simulink model "conmutador"  (Simulink 7.1)
settings: Solver=ode45  StartTime=0.0  StopTime=10000  RelTol=1e-3
values from neighbouring files (symbols this model uses):
  p = utilizacion(i)    [script_2x2.m]    (also in work.mat = 0.99)
libraries: simeventssink1 x8, simeventsrouting1 x8, simeventsqueue1 x4, simeventsgates1 x4, simeventsgenerators1 x4, simeventstiming1 x3, simeventsattributes1 x2, simeventsattributes2 x2, simeventsserver1 x2
settings Model: Creator=San  LastModifiedBy=EmP
settings DebuggingCC: SaveWithParameterizedLinksMsg=none  SignalResolutionControl=TryResolveAllWithWarning
settings GRTTargetCC: TargetFcnLib=ansi_tfl_tmw.mat
settings SimEventsCC: propLogEventsScheduled=0  propLogEventsExecuted=0  propLogDepartureEvents=0  propDisplayEventCalendar=0  propDiagAttribOutput=1  propDiagFcnCallOutput=1  propDiagStatOutput=0

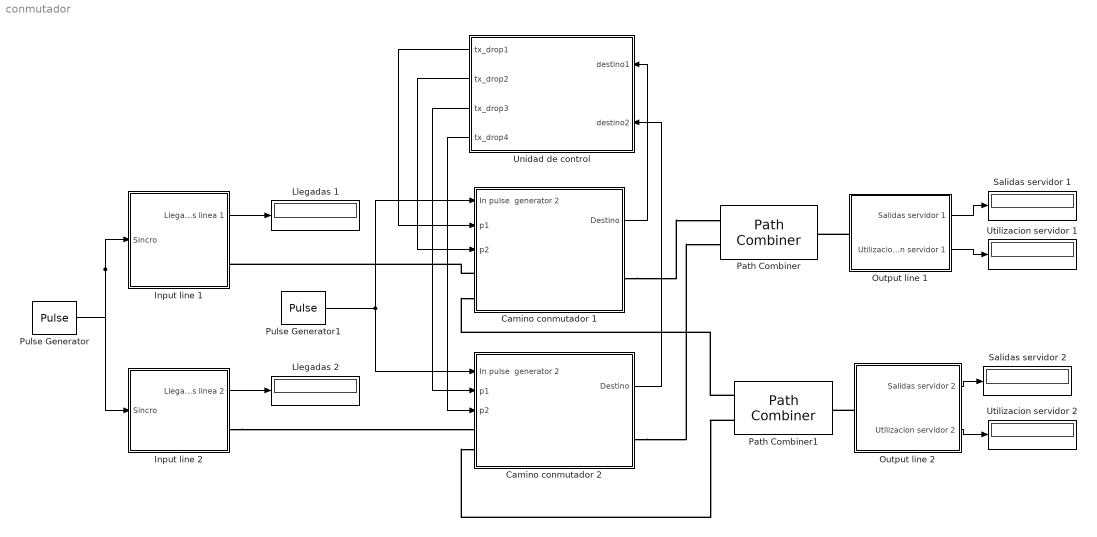
== system conmutador ==
  Camino conmutador 1 : Subsystem
  Camino conmutador 2 : Subsystem
  Input line 1 : Subsystem
  Input line 2 : Subsystem
  Llegadas 1 : Display
  Llegadas 2 : Display
  Output line 1 : Subsystem
  Output line 2 : Subsystem
  Path Combiner : simeventsrouting1/Path Combiner  Priority=1  SystemSampleTime=-1  NumberInputPorts=2  InputPortPrecedence=IN1 port  InitialSeed=45675  SpecifyEventPriority=off  PriorityPathCombinerPortPrecedenceSelection=4100  StatNumberDeparted=Off  StatLastArrivalPort=Off  EvaluatedNumPorts=2
  Path Combiner1 : simeventsrouting1/Path Combiner  Priority=1  SystemSampleTime=-1  NumberInputPorts=2  InputPortPrecedence=IN1 port  InitialSeed=45675  SpecifyEventPriority=off  PriorityPathCombinerPortPrecedenceSelection=4100  StatNumberDeparted=Off  StatLastArrivalPort=Off  EvaluatedNumPorts=2
  Pulse Generator : DiscretePulseGenerator  PulseType=Time based  Period=1  PulseWidth=50  SampleTime=1/10000
  Pulse Generator1 : DiscretePulseGenerator  PulseType=Time based  Period=1  PulseWidth=50  PhaseDelay=0.5  SampleTime=1/10000
  Salidas servidor 1 : Display
  Salidas servidor 2 : Display
  Unidad de control : Stateflow chart  Orientation=left
  Utilizacion servidor 1 : Display
  Utilizacion servidor 2 : Display
  wires:
  Pulse Generator/1 -> Input line 1/1(Sincro), Input line 2/1(Sincro)
  Camino conmutador 1/1(Destino) -> Unidad de control/1(destino1)
  Camino conmutador 2/1(Destino) -> Unidad de control/2(destino2)
  Unidad de control/1(tx_drop1) -> Camino conmutador 1/2(p1)
  Unidad de control/2(tx_drop2) -> Camino conmutador 1/3(p2)
  Unidad de control/3(tx_drop3) -> Camino conmutador 2/2(p1)
  Unidad de control/4(tx_drop4) -> Camino conmutador 2/3(p2)
  Pulse Generator1/1 -> Camino conmutador 1/1(In pulse  generator 2), Camino conmutador 2/1(In pulse  generator 2)
  Output line 1/2(Utilizacion servidor 1) -> Utilizacion servidor 1/1
  Output line 1/1(Salidas servidor 1) -> Salidas servidor 1/1
  Output line 2/1(Salidas servidor 2) -> Salidas servidor 2/1
  Output line 2/2(Utilizacion servidor 2) -> Utilizacion servidor 2/1
  Input line 2/1(Llegadas linea 2) -> Llegadas 2/1
  Input line 1/1(Llegadas linea 1) -> Llegadas 1/1
  connections:
  Camino conmutador 1/RConn1 -- Path Combiner/LConn1
  Camino conmutador 2/RConn1 -- Path Combiner/LConn2
  Path Combiner1/LConn2 -- Camino conmutador 2/LConn2
  Input line 2/RConn1 -- Camino conmutador 2/LConn1
  Camino conmutador 1/LConn1 -- Input line 1/RConn1
  Output line 1/LConn1 -- Path Combiner/RConn1
  Output line 2/LConn1 -- Path Combiner1/RConn1
  Path Combiner1/LConn1 -- Camino conmutador 1/LConn2

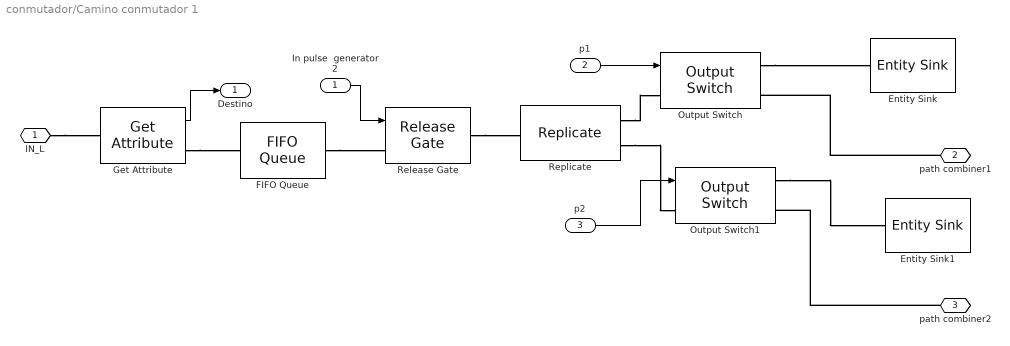
== system conmutador/Camino conmutador 1 ==
  In pulse  generator 2 : Inport  OutDataType=sfix(16)  OutScaling=2^0
  p1 : Inport  Port=2  OutDataType=sfix(16)  OutScaling=2^0
  p2 : Inport  Port=3  OutDataType=sfix(16)  OutScaling=2^0
  Entity Sink : simeventssink1/Entity Sink  Priority=1  SystemSampleTime=-1  AvailableForArrivals=on  StatNumberArrived=Off
  Entity Sink1 : simeventssink1/Entity Sink  Priority=1  SystemSampleTime=-1  AvailableForArrivals=on  StatNumberArrived=Off
  FIFO Queue : simeventsqueue1/FIFO Queue  Priority=1  SystemSampleTime=-1  Capacity=1  EnableTOPort=off  StatNumberDeparted=Off  StatNumberInBlock=Off  StatPendingEntity=Off  StatAverageWait=Off  StatAverageQueueLength=Off  StatNumberTimedout=Off
  Get Attribute : simeventsattributes1/Get Attribute  Priority=1  SystemSampleTime=-1  Attribute1To=On  Attribute1Name=Destino1  Attribute1Missing=Error  Attribute1DefaultValue=0  Attribute2To=Off  Attribute2Name=Attribute2  Attribute2Missing=Error  Attribute2DefaultValue=0  Attribute3To=Off  Attribute3Name=Attribute3  Attribute3Missing=Error  Attribute3DefaultValue=0  Attribute4To=Off  Attribute4Name=Attribute4  Attribute4Missing=Error  Attribute4DefaultValue=0  StatNumberDeparted=Off
  Output Switch : simeventsrouting1/Output Switch  Priority=1  SystemSampleTime=-1  NumberOutputPorts=2  SwitchingCriterion=From signal port p  InitialSeed=34567  AttributeName=Attribute1  InitialConditionsOpt=off  InitialConditions=1  EntityBufferOpt=off  SpecifyEventPriority=off  PriorityOutputSwitchSelectPort=4100  TimeoutPortOpt=off  StatNumberDeparted=Off  StatNumberTimedOut=Off  StatPendingEntity=Off  StatLastDeparturePort=Off  EvaluatedNumPorts=2
  Output Switch1 : simeventsrouting1/Output Switch  Priority=1  SystemSampleTime=-1  NumberOutputPorts=2  SwitchingCriterion=From signal port p  InitialSeed=34567  AttributeName=Attribute1  InitialConditionsOpt=off  InitialConditions=1  EntityBufferOpt=off  SpecifyEventPriority=off  PriorityOutputSwitchSelectPort=4100  TimeoutPortOpt=off  StatNumberDeparted=Off  StatNumberTimedOut=Off  StatPendingEntity=Off  StatLastDeparturePort=Off  EvaluatedNumPorts=2
  Release Gate : simeventsgates1/Release Gate  Priority=1  SystemSampleTime=-1  OpenGateUpon=Change in signal from port vc  SignalEdgeOption=Rising  SpecifyEventPriority=on  PriorityGateRelease=2200  StatNumberDeparted=Off
  Replicate : simeventsrouting1/Replicate  Priority=1  SystemSampleTime=-1  NumberOutputPorts=2  ReplicateEntityWhen=All entity output ports are not blocked  OutputPortPrecedence=OUT1 port  InitialSeed=56789  ActionUponBlocking=Discard entity  StatNumberArrived=Off  StatNumberDeparted=Off  EvaluatedNumPorts=2
  IN_L : PMIOPort  Port=1  Side=Left
  path combiner1 : PMIOPort  Orientation=left  Port=2  Side=Right
  path combiner2 : PMIOPort  Orientation=left  Port=3  Side=Left
  Destino : Outport  OutDataType=sfix(16)  OutScaling=2^0
  wires:
  p2/1 -> Output Switch1/1
  p1/1 -> Output Switch/1
  Get Attribute/1 -> Destino/1
  In pulse  generator 2/1 -> Release Gate/1
  connections:
  Release Gate/RConn1 -- Replicate/LConn1
  path combiner2/RConn1 -- Output Switch1/RConn2
  Replicate/RConn2 -- Output Switch1/LConn1
  path combiner1/RConn1 -- Output Switch/RConn2
  Replicate/RConn1 -- Output Switch/LConn1
  IN_L/RConn1 -- Get Attribute/LConn1
  FIFO Queue/RConn1 -- Release Gate/LConn1
  Get Attribute/RConn1 -- FIFO Queue/LConn1
  Output Switch1/RConn1 -- Entity Sink1/LConn1
  Output Switch/RConn1 -- Entity Sink/LConn1

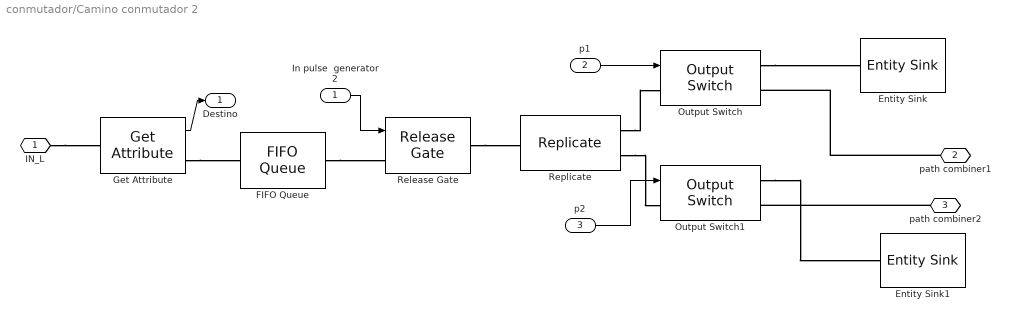
== system conmutador/Camino conmutador 2 ==
  In pulse  generator 2 : Inport  OutDataType=sfix(16)  OutScaling=2^0
  p1 : Inport  Port=2  OutDataType=sfix(16)  OutScaling=2^0
  p2 : Inport  Port=3  OutDataType=sfix(16)  OutScaling=2^0
  Entity Sink : simeventssink1/Entity Sink  Priority=1  SystemSampleTime=-1  AvailableForArrivals=on  StatNumberArrived=Off
  Entity Sink1 : simeventssink1/Entity Sink  Priority=1  SystemSampleTime=-1  AvailableForArrivals=on  StatNumberArrived=Off
  FIFO Queue : simeventsqueue1/FIFO Queue  Priority=1  SystemSampleTime=-1  Capacity=1  EnableTOPort=off  StatNumberDeparted=Off  StatNumberInBlock=Off  StatPendingEntity=Off  StatAverageWait=Off  StatAverageQueueLength=Off  StatNumberTimedout=Off
  Get Attribute : simeventsattributes1/Get Attribute  Priority=1  SystemSampleTime=-1  Attribute1To=On  Attribute1Name=Destino2  Attribute1Missing=Error  Attribute1DefaultValue=0  Attribute2To=Off  Attribute2Name=Attribute2  Attribute2Missing=Error  Attribute2DefaultValue=0  Attribute3To=Off  Attribute3Name=Attribute3  Attribute3Missing=Error  Attribute3DefaultValue=0  Attribute4To=Off  Attribute4Name=Attribute4  Attribute4Missing=Error  Attribute4DefaultValue=0  StatNumberDeparted=Off
  Output Switch : simeventsrouting1/Output Switch  Priority=1  SystemSampleTime=-1  NumberOutputPorts=2  SwitchingCriterion=From signal port p  InitialSeed=34567  AttributeName=Attribute1  InitialConditionsOpt=off  InitialConditions=1  EntityBufferOpt=off  SpecifyEventPriority=off  PriorityOutputSwitchSelectPort=4100  TimeoutPortOpt=off  StatNumberDeparted=Off  StatNumberTimedOut=Off  StatPendingEntity=Off  StatLastDeparturePort=Off  EvaluatedNumPorts=2
  Output Switch1 : simeventsrouting1/Output Switch  Priority=1  SystemSampleTime=-1  NumberOutputPorts=2  SwitchingCriterion=From signal port p  InitialSeed=34567  AttributeName=Attribute1  InitialConditionsOpt=off  InitialConditions=1  EntityBufferOpt=off  SpecifyEventPriority=off  PriorityOutputSwitchSelectPort=4100  TimeoutPortOpt=off  StatNumberDeparted=Off  StatNumberTimedOut=Off  StatPendingEntity=Off  StatLastDeparturePort=Off  EvaluatedNumPorts=2
  Release Gate : simeventsgates1/Release Gate  Priority=1  SystemSampleTime=-1  OpenGateUpon=Change in signal from port vc  SignalEdgeOption=Rising  SpecifyEventPriority=on  PriorityGateRelease=2200  StatNumberDeparted=Off
  Replicate : simeventsrouting1/Replicate  Priority=1  SystemSampleTime=-1  NumberOutputPorts=2  ReplicateEntityWhen=All entity output ports are not blocked  OutputPortPrecedence=OUT1 port  InitialSeed=56789  ActionUponBlocking=Discard entity  StatNumberArrived=Off  StatNumberDeparted=Off  EvaluatedNumPorts=2
  IN_L : PMIOPort  Port=1  Side=Left
  path combiner1 : PMIOPort  Orientation=left  Port=2  Side=Right
  path combiner2 : PMIOPort  Orientation=left  Port=3  Side=Left
  Destino : Outport  OutDataType=sfix(16)  OutScaling=2^0
  wires:
  p2/1 -> Output Switch1/1
  p1/1 -> Output Switch/1
  Get Attribute/1 -> Destino/1
  In pulse  generator 2/1 -> Release Gate/1
  connections:
  Release Gate/RConn1 -- Replicate/LConn1
  path combiner2/RConn1 -- Output Switch1/RConn2
  Replicate/RConn2 -- Output Switch1/LConn1
  path combiner1/RConn1 -- Output Switch/RConn2
  Replicate/RConn1 -- Output Switch/LConn1
  IN_L/RConn1 -- Get Attribute/LConn1
  FIFO Queue/RConn1 -- Release Gate/LConn1
  Get Attribute/RConn1 -- FIFO Queue/LConn1
  Output Switch1/RConn1 -- Entity Sink1/LConn1
  Output Switch/RConn1 -- Entity Sink/LConn1

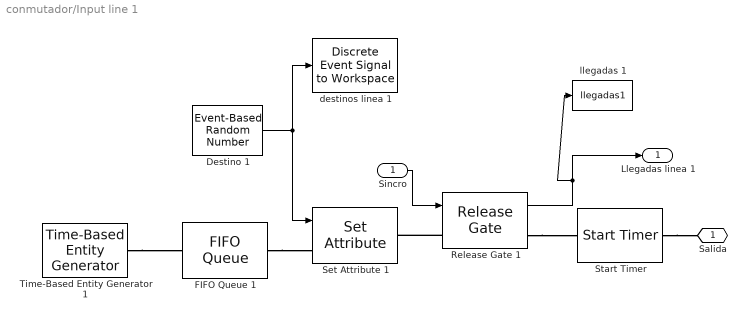
== system conmutador/Input line 1 ==
  Sincro : Inport
  Destino 1 : simeventsgenerators1/Signal Generators/Event-Based Random Number  SystemSampleTime=-1  distribution=Arbitrary discrete  meanExp=1  minUnif=1  maxUnif=2  pOneBern=0.25  pSuccessBino=0.5  numTrialBino=1  meanNorm=0  stdNorm=1  minTri=1  maxTri=3  modeTri=2  thresholdLogn=0  scaleLogn=1  shapeLogn=1  pSuccessGeo=0.5  meanPoiss=1  thresholdLogl=0  scaleLogl=1  thresholdGam=0  scaleGam=1  shapeGam=1  minBeta=0  maxBeta=1  shape1Beta=1  shape2Beta=1  minUnid=1  maxUnid=2  numValueUnid=2  thresholdWbl=0  scaleWbl=1  shapeWbl=1  valueVecCont=[0 1]  cdfVecCont=[0 1]  valueVecDisc=[0 1 2]  probVecDisc=[(1-p) p/2 p/2]  seed=875632  IsProcessed=on  isConnected=1
  FIFO Queue 1 : simeventsqueue1/FIFO Queue  Priority=1  SystemSampleTime=-1  Capacity=inf  EnableTOPort=off  StatNumberDeparted=Off  StatNumberInBlock=Off  StatPendingEntity=Off  StatAverageWait=Off  StatAverageQueueLength=Off  StatNumberTimedout=Off
  Release Gate 1 : simeventsgates1/Release Gate  Priority=1  SystemSampleTime=-1  OpenGateUpon=Change in signal from port vc  SignalEdgeOption=Rising  SpecifyEventPriority=off  PriorityGateRelease=2200  StatNumberDeparted=On
  Set Attribute 1 : simeventsattributes2/Set Attribute  Priority=1  DialogController=des_ddg_create  DialogControllerArgs=DataTag19  SystemSampleTime=-1  AttributeFrom=Signal port  AttributeName=Destino1  AttributeTreatAsVector=1  AttributeValue=1  AttributeCreate=on  StatNumberDeparted=Off  EvaluatedAttributeValue={[]}
  Start Timer : simeventstiming1/Start Timer  Priority=0  SystemSampleTime=-1  TimerTag=retardo  TimerStartedOption=Warn and continue  StatNumberDeparted=Off
  Time-Based Entity Generator 1 : simeventsgenerators1/Entity Generators/Time-Based Entity Generator  Priority=1  DialogController=des_ddg_create  DialogControllerArgs=DataTag22  SystemSampleTime=-1  GenerateEntitiesUpon=Intergeneration time from dialog  Distribution=Constant  Minimum=0  Maximum=1  Mean=1  InitialSeed=12345  Period=0.5  PriorityEntityGeneration=300  GenerateEntityAtSimulationStart=on  ResponseWhenBlocked=Pause generation  ResponseWhenUnblocked=Immediate restart  EntityType=Blank  StatNumberDeparted=Off  StatPendingEntity=Off  StatAverageIntergenerationTime=Off
  destinos linea 1 : simeventssink1/Discrete Event Signal to Workspace  SystemSampleTime=-1  VariableName=destinos1  SaveFormat=Array  IsMonitorOnly=off
  llegadas 1 : ToWorkspace  VariableName=llegadas1  SampleTime=10000  SaveFormat=Array
  Salida : PMIOPort  Orientation=left  Port=1  Side=Right
  Llegadas linea 1 : Outport  OutDataType=sfix(16)  OutScaling=2^0
  wires:
  Destino 1/1 -> Set Attribute 1/1, destinos linea 1/1
  Sincro/1 -> Release Gate 1/1
  Release Gate 1/1 -> Llegadas linea 1/1, llegadas 1/1
  connections:
  Time-Based Entity Generator 1/RConn1 -- FIFO Queue 1/LConn1
  FIFO Queue 1/RConn1 -- Set Attribute 1/LConn1
  Release Gate 1/LConn1 -- Set Attribute 1/RConn1
  Start Timer/RConn1 -- Salida/RConn1
  Release Gate 1/RConn1 -- Start Timer/LConn1

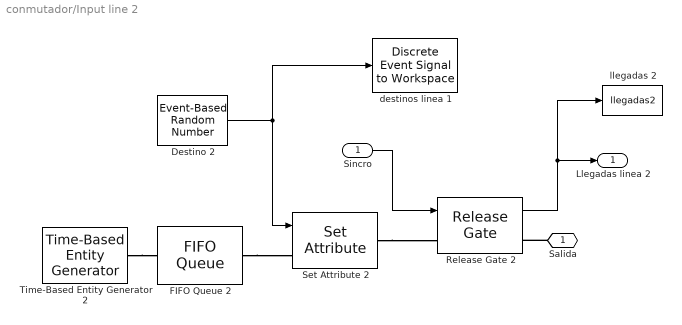
== system conmutador/Input line 2 ==
  Sincro : Inport
  Destino 2 : simeventsgenerators1/Signal Generators/Event-Based Random Number  SystemSampleTime=-1  distribution=Arbitrary discrete  meanExp=1  minUnif=1  maxUnif=1  pOneBern=0.25  pSuccessBino=0.5  numTrialBino=1  meanNorm=0  stdNorm=1  minTri=1  maxTri=3  modeTri=2  thresholdLogn=0  scaleLogn=1  shapeLogn=1  pSuccessGeo=0.5  meanPoiss=1  thresholdLogl=0  scaleLogl=1  thresholdGam=0  scaleGam=1  shapeGam=1  minBeta=0  maxBeta=1  shape1Beta=1  shape2Beta=1  minUnid=1  maxUnid=2  numValueUnid=2  thresholdWbl=0  scaleWbl=1  shapeWbl=1  valueVecCont=[0 1]  cdfVecCont=[0 1]  valueVecDisc=[0 1 2]  probVecDisc=[(1-p) p/2 p/2]  seed=0964  IsProcessed=on  isConnected=1
  FIFO Queue 2 : simeventsqueue1/FIFO Queue  Priority=1  SystemSampleTime=-1  Capacity=1000000  EnableTOPort=off  StatNumberDeparted=Off  StatNumberInBlock=Off  StatPendingEntity=Off  StatAverageWait=Off  StatAverageQueueLength=Off  StatNumberTimedout=Off
  Release Gate 2 : simeventsgates1/Release Gate  Priority=1  SystemSampleTime=-1  OpenGateUpon=Change in signal from port vc  SignalEdgeOption=Rising  SpecifyEventPriority=off  PriorityGateRelease=2200  StatNumberDeparted=On
  Set Attribute 2 : simeventsattributes2/Set Attribute  Priority=1  DialogController=des_ddg_create  DialogControllerArgs=DataTag26  SystemSampleTime=-1  AttributeFrom=Signal port  AttributeName=Destino2  AttributeTreatAsVector=1  AttributeValue=1  AttributeCreate=on  StatNumberDeparted=Off  EvaluatedAttributeValue={[]}
  Time-Based Entity Generator 2 : simeventsgenerators1/Entity Generators/Time-Based Entity Generator  Priority=1  DialogController=des_ddg_create  DialogControllerArgs=DataTag28  SystemSampleTime=-1  GenerateEntitiesUpon=Intergeneration time from dialog  Distribution=Constant  Minimum=0  Maximum=1  Mean=1  InitialSeed=543541  Period=1  PriorityEntityGeneration=300  GenerateEntityAtSimulationStart=on  ResponseWhenBlocked=Pause generation  ResponseWhenUnblocked=Immediate restart  EntityType=Blank  StatNumberDeparted=Off  StatPendingEntity=Off  StatAverageIntergenerationTime=Off
  destinos linea 1 : simeventssink1/Discrete Event Signal to Workspace  SystemSampleTime=-1  VariableName=destinos2  SaveFormat=Array  IsMonitorOnly=off
  llegadas 2 : ToWorkspace  VariableName=llegadas2  SampleTime=10000  SaveFormat=Array
  Salida : PMIOPort  Orientation=left  Port=1  Side=Right
  Llegadas linea 2 : Outport  OutDataType=sfix(16)  OutScaling=2^0
  wires:
  Destino 2/1 -> Set Attribute 2/1, destinos linea 1/1
  Sincro/1 -> Release Gate 2/1
  Release Gate 2/1 -> Llegadas linea 2/1, llegadas 2/1
  connections:
  Time-Based Entity Generator 2/RConn1 -- FIFO Queue 2/LConn1
  Set Attribute 2/RConn1 -- Release Gate 2/LConn1
  Salida/RConn1 -- Release Gate 2/RConn1
  FIFO Queue 2/RConn1 -- Set Attribute 2/LConn1

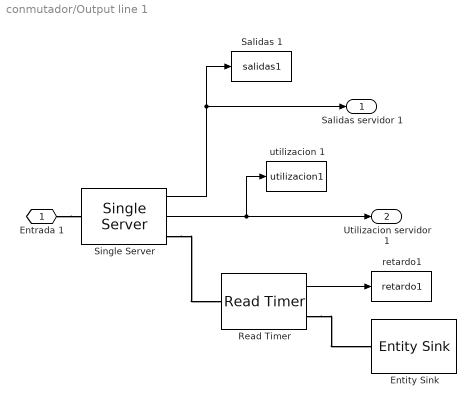
== system conmutador/Output line 1 ==
  Entity Sink : simeventssink1/Entity Sink  Priority=1  SystemSampleTime=-1  AvailableForArrivals=on  StatNumberArrived=Off
  Read Timer : simeventstiming1/Read Timer  Priority=0  SystemSampleTime=-1  TimerTag=retardo  TimerModeOption=Ignore  TimerStop=off  StatNumberDeparted=Off  StatTimerNumberDeparted=Off  StatTimeElapsed=Off  StatAverageTimeElapsed=On
  Salidas 1 : ToWorkspace  VariableName=salidas1  SampleTime=10000  SaveFormat=Array
  Single Server : simeventsserver1/Single Server  Priority=1  SystemSampleTime=-1  ServiceTimeFrom=Dialog  ServiceTime=0.99999  AttributeName=ServiceTime  PriorityServiceCompletion=500  PermitPreemption=off  SortingAttributeName=PriorityAttributeName  SortingDirection=Ascending  WriteToAttribute=off  ResidualAttributeName=ResidualServiceTime  CreateAttribute=on  EnableTOPort=off  StatNumberDeparted=On  StatNumberInBlock=Off  StatNumberPreempted=Off  StatPendingEntity=Off  StatAverageWait=Off  StatUtilization=On  StatNumberTimedout=Off
  retardo1 : ToWorkspace  VariableName=retardo1  SampleTime=10000  SaveFormat=Array
  utilizacion 1 : ToWorkspace  VariableName=utilizacion1  SampleTime=10000  SaveFormat=Array
  Entrada 1 : PMIOPort  Port=1  Side=Left
  Salidas servidor 1 : Outport  OutDataType=sfix(16)  OutScaling=2^0
  Utilizacion servidor 1 : Outport  Port=2  OutDataType=sfix(16)  OutScaling=2^0
  wires:
  Single Server/1 -> Salidas 1/1, Salidas servidor 1/1
  Single Server/2 -> Utilizacion servidor 1/1, utilizacion 1/1
  Read Timer/1 -> retardo1/1
  connections:
  Entrada 1/RConn1 -- Single Server/LConn1
  Read Timer/RConn1 -- Entity Sink/LConn1
  Single Server/RConn1 -- Read Timer/LConn1

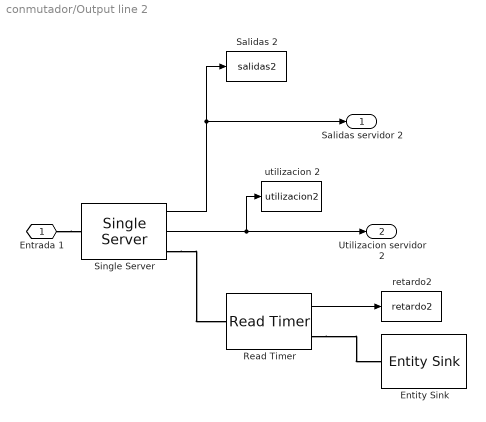
== system conmutador/Output line 2 ==
  Entity Sink : simeventssink1/Entity Sink  Priority=1  SystemSampleTime=-1  AvailableForArrivals=on  StatNumberArrived=Off
  Read Timer : simeventstiming1/Read Timer  Priority=0  SystemSampleTime=-1  TimerTag=retardo  TimerModeOption=Ignore  TimerStop=off  StatNumberDeparted=Off  StatTimerNumberDeparted=Off  StatTimeElapsed=Off  StatAverageTimeElapsed=On
  Salidas 2 : ToWorkspace  VariableName=salidas2  SampleTime=10000  SaveFormat=Array
  Single Server : simeventsserver1/Single Server  Priority=1  SystemSampleTime=-1  ServiceTimeFrom=Dialog  ServiceTime=0.99999  AttributeName=ServiceTime  PriorityServiceCompletion=500  PermitPreemption=off  SortingAttributeName=PriorityAttributeName  SortingDirection=Ascending  WriteToAttribute=off  ResidualAttributeName=ResidualServiceTime  CreateAttribute=on  EnableTOPort=off  StatNumberDeparted=On  StatNumberInBlock=Off  StatNumberPreempted=Off  StatPendingEntity=Off  StatAverageWait=Off  StatUtilization=On  StatNumberTimedout=Off
  retardo2 : ToWorkspace  VariableName=retardo2  SampleTime=10000  SaveFormat=Array
  utilizacion 2 : ToWorkspace  VariableName=utilizacion2  SampleTime=10000  SaveFormat=Array
  Entrada 1 : PMIOPort  Port=1  Side=Left
  Salidas servidor 2 : Outport  OutDataType=sfix(16)  OutScaling=2^0
  Utilizacion servidor 2 : Outport  Port=2  OutDataType=sfix(16)  OutScaling=2^0
  wires:
  Single Server/1 -> Salidas 2/1, Salidas servidor 2/1
  Single Server/2 -> Utilizacion servidor 2/1, utilizacion 2/1
  Read Timer/1 -> retardo2/1
  connections:
  Entrada 1/RConn1 -- Single Server/LConn1
  Read Timer/RConn1 -- Entity Sink/LConn1
  Single Server/RConn1 -- Read Timer/LConn1

== matlab function Unidad de control ==
  data: destino1 input double; tx_drop1 output double; destino2 input double; tx_drop2 output double; tx_drop3 output double; tx_drop4 output double
function [tx_drop1, tx_drop2,tx_drop3,tx_drop4] = port_selection_line(destino1,destino2)
 
%matriz de conmutacion: filas=entradas, columnas=salidas
matriz_com=ones(2,2);           
 
%vector de destinos de cada entrada
destinos=[destino1, destino2];      
 
%Rellenamos la matriz de conmutación con los destinos correspondientes
for i=1:1:length(destinos)
      matriz_com(i,:)=asignar_puertos(destinos(i)); 
end
 
%Comprobamos las columnas de la matriz. Si en una columna hay más de un elemento que sea un 2-> conflicto
for j=1:length(matriz_com(1,:))
     entradas_en_conflicto=zeros(1,length(destinos));%Vector que almacena aquellas entradas que generan el conflicto
     %verificamos las entradas que quieren salir por la salida j
     for i=1:length(matriz_com(:,1))
         if matriz_com(i,j)==2
            entradas_en_conflicto(i)=1;                     
         end    
     end  
 
     %Comprobamos si hay conflicto
     if sum(entradas_en_conflicto)>1                         
        %Resolvemos el conflicto
        matriz_com(:,j)=resolver_conflicto(entradas_en_conflicto);
     end
end
 
%Asignamos las señales tx_drop a sus valores correspondientes según la matriz de conmutación
tx_drop1=matriz_com(1,1);
tx_drop2=matriz_com(1,2);
tx_drop3=matriz_com(2,1);
tx_drop4=matriz_com(2,2);
 
 
%%%%%%%% Funciones adicionales
%Introduce un 2 (la entrada quiere salir por la fila relativa a esa columna) en la columna
%correspondiente de la matriz para una entrada.
function [puertos]=asignar_puertos(destino)
    puertos=ones(1,2);
    if destino~=0%Si es cero, el paquete debe descartarse -> se deja en la matriz un 1
        puertos(destino)=2;
    end
 
%Elige de forma aleatoria una entrada para resolver un conflicto y devuelve la columna que debería
%tener la matriz de conmutación tras la resolución del mismo.
function [columna]=resolver_conflicto(entradas)
    cont=0;
    ent=0;
    columna=ones(2,1);
    aux=sum(entradas);%Sumamos el vector de entradas para saber cuantas líneas hay en conflicto
    seleccion=ceil(aux*rand(1));%Elegimos de forma aleatoria una de las entradas
    
    for i=1:length(entradas)
        if entradas(i)==1
            cont=cont+1;
            if cont==seleccion
            ent=i;
            end
        end
    end
    columna(ent)=2; %Ponemos un 2 en la línea que finalmente sale ganadora del conflicto y dejamos las demás a 1
